simulink model "friction_model"  (R2021a)
settings: Solver=VariableStepAuto  StartTime=0.0  StopTime=10.0  RelTol=1e-3
InitFcn:
  | Jm=100;
  | fric_gear=1;
settings Model: Creator=גבי דוידוב  LastModifiedBy=גבי דוידוב

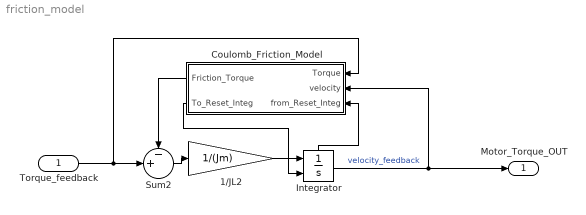
== system friction_model ==
  Torque_feedback : Inport
  1/JL2 : Gain  Gain=1/(Jm)  SaturateOnIntegerOverflow=on  OutDataTypeStr=Inherit: Same as input  ParamDataTypeStr=Inherit: Same as input
  Coulomb_Friction_Model : Subsystem
  Integrator : Integrator  ExternalReset=rising  ShowStatePort=on
  Sum2 : Sum  Inputs=-+|  SaturateOnIntegerOverflow=on
  Motor_Torque_OUT : Outport
  wires:
  Coulomb_Friction_Model/1(Friction_Torque) -> Sum2/1
  Integrator/State -> Coulomb_Friction_Model/3(from_Reset_Integ)
  Coulomb_Friction_Model/2(To_Reset_Integ) -> Integrator/2
  Torque_feedback/1 -> Coulomb_Friction_Model/1(Torque), Sum2/2
  1/JL2/1 -> Integrator/1
  Integrator/1 -> Motor_Torque_OUT/1, Coulomb_Friction_Model/2(velocity)  "velocity_feedback"
  Sum2/1 -> 1/JL2/1

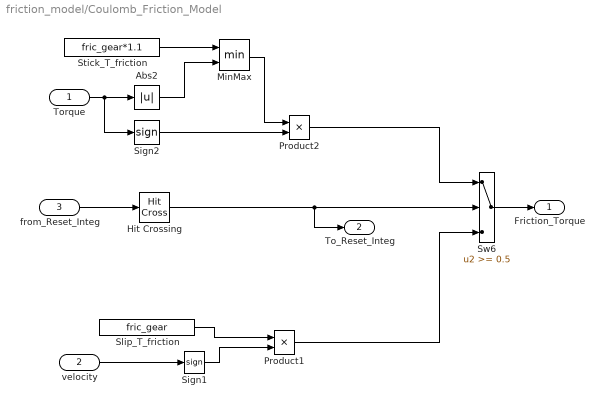
== system friction_model/Coulomb_Friction_Model ==
  Torque : Inport
  velocity : Inport  Port=2
  from_Reset_Integ : Inport  Port=3
  Abs2 : Abs
  Hit Crossing : HitCross  ZeroCross=off
  MinMax : MinMax  Inputs=2
  Product1 : Product  RndMeth=Zero
  Product2 : Product  RndMeth=Zero
  Sign1 : Signum  ZeroCross=off
  Sign2 : Signum  ZeroCross=off
  Slip_T_friction : Constant  Value=fric_gear
  Stick_T_friction : Constant  Value=fric_gear*1.1
  Sw6 : Switch  Threshold=0.5  SaturateOnIntegerOverflow=on  InputSameDT=on
  Friction_Torque : Outport
  To_Reset_Integ : Outport  Port=2
  wires:
  Torque/1 -> Abs2/1, Sign2/1
  Sw6/1 -> Friction_Torque/1
  velocity/1 -> Sign1/1
  Sign1/1 -> Product1/2
  Product1/1 -> Sw6/3
  Hit Crossing/1 -> To_Reset_Integ/1, Sw6/2
  from_Reset_Integ/1 -> Hit Crossing/1
  Sign2/1 -> Product2/2
  Stick_T_friction/1 -> MinMax/1
  Abs2/1 -> MinMax/2
  MinMax/1 -> Product2/1
  Product2/1 -> Sw6/1
  Slip_T_friction/1 -> Product1/1
